simulink model "Linear_model"  (R2025b)
settings: Solver=VariableStepAuto  StartTime=0.0  StopTime=10.0  RelTol=1e-3
values from neighbouring files (symbols this model uses):
  A1 = [0, 1; 0, 0]    [linear_pole_placemet - Main Sim.m]    (also in non_linear_pole_placemet - Main Sim.m)
  A2 = [0, 0, 1, 0; 0, 0, 0, 1; 0, g, 0, 0; 0, 0, 0, 0]    [linear_pole_placemet - Main Sim.m]    (also in non_linear_pole_placemet - Main Sim.m)
  A3 = [0, 0, 1, 0; 0, 0, 0, 1; 0, -g, 0, 0; 0, 0, 0, 0]    [linear_pole_placemet - Main Sim.m]    (also in non_linear_pole_placemet - Main Sim.m)
  A4 = [0, 1; 0, 0]    [linear_pole_placemet - Main Sim.m]    (also in non_linear_pole_placemet - Main Sim.m)
  B1 = [0; 1/m]    [linear_pole_placemet - Main Sim.m]    (also in non_linear_pole_placemet - Main Sim.m)
  B2 = [0; 0; 0; 1/J11]    [linear_pole_placemet - Main Sim.m]    (also in non_linear_pole_placemet - Main Sim.m)
  B3 = [0; 0; 0; 1/J22]    [linear_pole_placemet - Main Sim.m]    (also in non_linear_pole_placemet - Main Sim.m)
  B4 = [0; 1/J33]    [linear_pole_placemet - Main Sim.m]    (also in non_linear_pole_placemet - Main Sim.m)
  C1 = eye(2)    [linear_pole_placemet - Main Sim.m]    (also in non_linear_pole_placemet - Main Sim.m)
  C2 = eye(4)    [linear_pole_placemet - Main Sim.m]    (also in non_linear_pole_placemet - Main Sim.m)
  C3 = eye(4)    [linear_pole_placemet - Main Sim.m]    (also in non_linear_pole_placemet - Main Sim.m)
  C4 = eye(2)    [linear_pole_placemet - Main Sim.m]    (also in non_linear_pole_placemet - Main Sim.m)
  D1 = zeros(2, 1)    [linear_pole_placemet - Main Sim.m]    (also in non_linear_pole_placemet - Main Sim.m)
  D2 = zeros(4, 1)    [linear_pole_placemet - Main Sim.m]    (also in non_linear_pole_placemet - Main Sim.m)
  D3 = zeros(4, 1)    [linear_pole_placemet - Main Sim.m]    (also in non_linear_pole_placemet - Main Sim.m)
  D4 = zeros(2, 1)    [linear_pole_placemet - Main Sim.m]    (also in non_linear_pole_placemet - Main Sim.m)
  K1 = real(ackermann(A1, B1, poles1))    [linear_pole_placemet - Main Sim.m]    (also in non_linear_pole_placemet - Main Sim.m)
  K2 = real(ackermann(A2, B2, poles2))    [linear_pole_placemet - Main Sim.m]    (also in non_linear_pole_placemet - Main Sim.m)
  K3 = real(ackermann(A3, B3, poles3))    [linear_pole_placemet - Main Sim.m]    (also in non_linear_pole_placemet - Main Sim.m)
  K4 = real(ackermann(A4, B4, poles4))    [linear_pole_placemet - Main Sim.m]    (also in non_linear_pole_placemet - Main Sim.m)
  ki1 = prefilter(A1, B1, C1(1,:), K1)    [linear_pole_placemet - Main Sim.m]    (also in non_linear_pole_placemet - Main Sim.m)
  ki2 = prefilter(A2, B2, C2(1,:), K2)    [linear_pole_placemet - Main Sim.m]    (also in non_linear_pole_placemet - Main Sim.m)
  ki3 = prefilter(A3, B3, C3(1,:), K3)    [linear_pole_placemet - Main Sim.m]    (also in non_linear_pole_placemet - Main Sim.m)
  ki4 = prefilter(A4, B4, C4(1,:), K4)    [linear_pole_placemet - Main Sim.m]    (also in non_linear_pole_placemet - Main Sim.m)
  phi_ref = 0.5    [linear_pole_placemet - Main Sim.m]    (also in non_linear_pole_placemet - Main Sim.m)
  x_ref = 2    [linear_pole_placemet - Main Sim.m]    (also in non_linear_pole_placemet - Main Sim.m)
  y_ref = 1    [linear_pole_placemet - Main Sim.m]    (also in non_linear_pole_placemet - Main Sim.m)
  z_ref = 4    [linear_pole_placemet - Main Sim.m]    (also in non_linear_pole_placemet - Main Sim.m)
settings Model: Creator=joaom  LastModifiedBy=joaom
settings DataIOCC: SaveFormat=Array

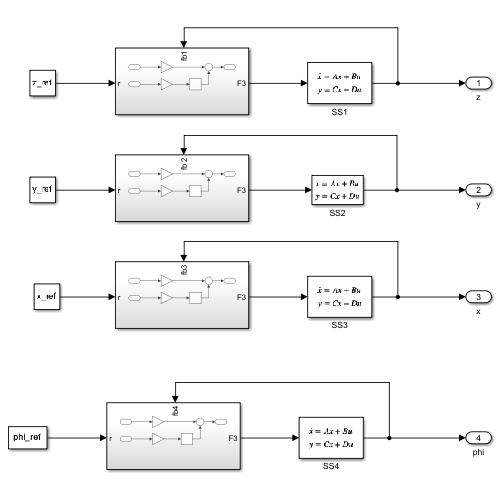
[thumbnail: Simulink's stored preview of the top-level diagram]
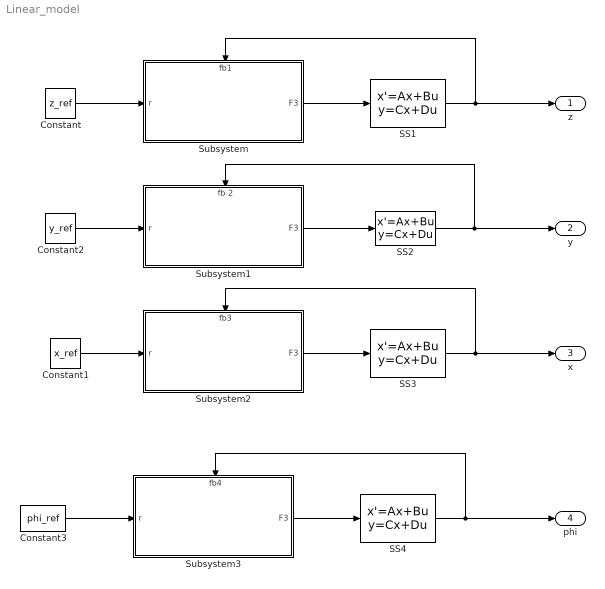
== system Linear_model ==
  Constant : Constant  Value=z_ref
  Constant1 : Constant  Value=x_ref
  Constant2 : Constant  Value=y_ref
  Constant3 : Constant  Value=phi_ref
  SS1 : StateSpace  A=A1  B=B1  C=C1  D=D1  InitialCondition=[0.5;0]
  SS2 : StateSpace  A=A2  B=B2  C=C2  D=D2  InitialCondition=0
  SS3 : StateSpace  A=A3  B=B3  C=C3  D=D3  InitialCondition=[1;0.1;0;0]
  SS4 : StateSpace  A=A4  B=B4  C=C4  D=D4  InitialCondition=[0.1;0]
  Subsystem : Subsystem
      settings: PortSchema="{\"entries\":[{\"content\":{\"sides\":[{\"content\":{\"connectorIds\":[\"In1\"]},\"type\":\"ConnectorPlacement.EquallySpacedRectSide\",\"uuid\":\"b3654a7f-5063-48c0-9b36-91e0db63b0ba\"},{\"content\":{\"connectorIds\":[\"Out1\"],\"side\":\"RIGHT\"},\"type\":\"ConnectorPlacement.EquallySpacedRectSide\",\"uuid\":\"218488d6-68f2-41aa-8299-f3fb09ba40d8\"},{\"content\":{\"connectorIds\":[\"In2\"],\"side\":\"TOP\"},\"type\":\"ConnectorPlacement.EquallySpacedRectSide\",\"uuid\":\"ffca8f5f-99ce-4cfe-b848-505d5918397a\"},{\"content\":{\"side\":\"BOTTOM\"},\"type\":\"ConnectorPlacement.EquallySpacedRectSide\",\"uuid\":\"0ee1b0b7-fa1d-4d2f-b721-1db90edeb8b7\"}]},\"type\":\"ConnectorPlacement.EquallySpacedConnector\",\"uuid\":\"97e1b17e-acc2-4e54-bcf8-8316abbe6834\"}],\"packageUris\":[\"http://schema.mathworks.com/mf0/Connector/R2020b\"],\"version\":\"1.0\"}"
  Subsystem1 : Subsystem
      settings: PortSchema="{\"entries\":[{\"content\":{\"sides\":[{\"content\":{\"connectorIds\":[\"In1\"]},\"type\":\"ConnectorPlacement.EquallySpacedRectSide\",\"uuid\":\"b3654a7f-5063-48c0-9b36-91e0db63b0ba\"},{\"content\":{\"connectorIds\":[\"Out1\"],\"side\":\"RIGHT\"},\"type\":\"ConnectorPlacement.EquallySpacedRectSide\",\"uuid\":\"218488d6-68f2-41aa-8299-f3fb09ba40d8\"},{\"content\":{\"connectorIds\":[\"In2\"],\"side\":\"TOP\"},\"type\":\"ConnectorPlacement.EquallySpacedRectSide\",\"uuid\":\"ffca8f5f-99ce-4cfe-b848-505d5918397a\"},{\"content\":{\"side\":\"BOTTOM\"},\"type\":\"ConnectorPlacement.EquallySpacedRectSide\",\"uuid\":\"0ee1b0b7-fa1d-4d2f-b721-1db90edeb8b7\"}]},\"type\":\"ConnectorPlacement.EquallySpacedConnector\",\"uuid\":\"97e1b17e-acc2-4e54-bcf8-8316abbe6834\"}],\"packageUris\":[\"http://schema.mathworks.com/mf0/Connector/R2020b\"],\"version\":\"1.0\"}"
  Subsystem2 : Subsystem
      settings: PortSchema="{\"entries\":[{\"content\":{\"sides\":[{\"content\":{\"connectorIds\":[\"In1\"]},\"type\":\"ConnectorPlacement.EquallySpacedRectSide\",\"uuid\":\"b3654a7f-5063-48c0-9b36-91e0db63b0ba\"},{\"content\":{\"connectorIds\":[\"Out1\"],\"side\":\"RIGHT\"},\"type\":\"ConnectorPlacement.EquallySpacedRectSide\",\"uuid\":\"218488d6-68f2-41aa-8299-f3fb09ba40d8\"},{\"content\":{\"connectorIds\":[\"In2\"],\"side\":\"TOP\"},\"type\":\"ConnectorPlacement.EquallySpacedRectSide\",\"uuid\":\"ffca8f5f-99ce-4cfe-b848-505d5918397a\"},{\"content\":{\"side\":\"BOTTOM\"},\"type\":\"ConnectorPlacement.EquallySpacedRectSide\",\"uuid\":\"0ee1b0b7-fa1d-4d2f-b721-1db90edeb8b7\"}]},\"type\":\"ConnectorPlacement.EquallySpacedConnector\",\"uuid\":\"97e1b17e-acc2-4e54-bcf8-8316abbe6834\"}],\"packageUris\":[\"http://schema.mathworks.com/mf0/Connector/R2020b\"],\"version\":\"1.0\"}"
  Subsystem3 : Subsystem
      settings: PortSchema="{\"entries\":[{\"content\":{\"sides\":[{\"content\":{\"connectorIds\":[\"In1\"]},\"type\":\"ConnectorPlacement.EquallySpacedRectSide\",\"uuid\":\"b3654a7f-5063-48c0-9b36-91e0db63b0ba\"},{\"content\":{\"connectorIds\":[\"Out1\"],\"side\":\"RIGHT\"},\"type\":\"ConnectorPlacement.EquallySpacedRectSide\",\"uuid\":\"218488d6-68f2-41aa-8299-f3fb09ba40d8\"},{\"content\":{\"connectorIds\":[\"In2\"],\"side\":\"TOP\"},\"type\":\"ConnectorPlacement.EquallySpacedRectSide\",\"uuid\":\"ffca8f5f-99ce-4cfe-b848-505d5918397a\"},{\"content\":{\"side\":\"BOTTOM\"},\"type\":\"ConnectorPlacement.EquallySpacedRectSide\",\"uuid\":\"0ee1b0b7-fa1d-4d2f-b721-1db90edeb8b7\"}]},\"type\":\"ConnectorPlacement.EquallySpacedConnector\",\"uuid\":\"97e1b17e-acc2-4e54-bcf8-8316abbe6834\"}],\"packageUris\":[\"http://schema.mathworks.com/mf0/Connector/R2020b\"],\"version\":\"1.0\"}"
  z : Outport
  y : Outport  Port=2
  x : Outport  Port=3
  phi : Outport  Port=4
  wires:
  Constant/1 -> Subsystem/1(r)
  Subsystem/1(F3) -> SS1/1
  SS1/1 -> Subsystem/2(fb1), z/1
  Constant2/1 -> Subsystem1/1(r)
  Subsystem1/1(F3) -> SS2/1
  SS3/1 -> Subsystem2/2(fb3), x/1
  Constant1/1 -> Subsystem2/1(r)
  Subsystem2/1(F3) -> SS3/1
  SS4/1 -> Subsystem3/2(fb4), phi/1
  Constant3/1 -> Subsystem3/1(r)
  Subsystem3/1(F3) -> SS4/1
  SS2/1 -> y/1, Subsystem1/2(fb 2)

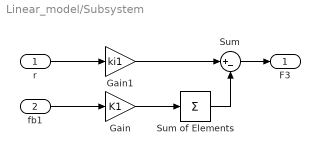
== system Linear_model/Subsystem ==
  r : Inport
  fb1 : Inport  Port=2
  Gain : Gain  Gain=K1
  Gain1 : Gain  Gain=ki1
  Sum : Sum  Inputs=|+-
  Sum of Elements : Sum  Inputs=+
  F3 : Outport
  wires:
  r/1 -> Gain1/1
  Gain1/1 -> Sum/1
  Sum/1 -> F3/1
  fb1/1 -> Gain/1
  Gain/1 -> Sum of Elements/1
  Sum of Elements/1 -> Sum/2

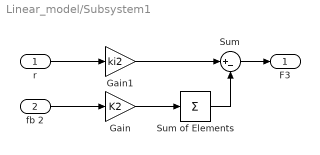
== system Linear_model/Subsystem1 ==
  r : Inport
  fb 2 : Inport  Port=2
  Gain : Gain  Gain=K2
  Gain1 : Gain  Gain=ki2
  Sum : Sum  Inputs=|+-
  Sum of Elements : Sum  Inputs=+
  F3 : Outport
  wires:
  r/1 -> Gain1/1
  Gain1/1 -> Sum/1
  Sum/1 -> F3/1
  fb 2/1 -> Gain/1
  Gain/1 -> Sum of Elements/1
  Sum of Elements/1 -> Sum/2

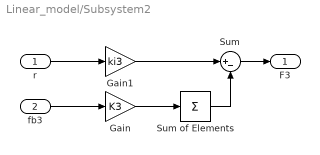
== system Linear_model/Subsystem2 ==
  r : Inport
  fb3 : Inport  Port=2
  Gain : Gain  Gain=K3
  Gain1 : Gain  Gain=ki3
  Sum : Sum  Inputs=|+-
  Sum of Elements : Sum  Inputs=+
  F3 : Outport
  wires:
  r/1 -> Gain1/1
  Gain1/1 -> Sum/1
  Sum/1 -> F3/1
  fb3/1 -> Gain/1
  Gain/1 -> Sum of Elements/1
  Sum of Elements/1 -> Sum/2

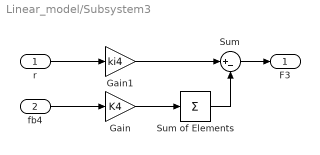
== system Linear_model/Subsystem3 ==
  r : Inport
  fb4 : Inport  Port=2
  Gain : Gain  Gain=K4
  Gain1 : Gain  Gain=ki4
  Sum : Sum  Inputs=|+-
  Sum of Elements : Sum  Inputs=+
  F3 : Outport
  wires:
  r/1 -> Gain1/1
  Gain1/1 -> Sum/1
  Sum/1 -> F3/1
  fb4/1 -> Gain/1
  Gain/1 -> Sum of Elements/1
  Sum of Elements/1 -> Sum/2
